simulink model "FullRect_verify"  (R2022b)
settings: Solver=VariableStepAuto  StartTime=0.0  StopTime=0.001  RelTol=1e-3
InitFcn:
  | rng("shuffle");
  | %seed = round(rand(1)*1000);
  | seed = 100;
StopFcn:
  | writematrix(out.input, "C:\Users\dmesenge\Documents\School\PattRecNN\Project\models\FullRect_test_inputs.csv")
  | writematrix(out.actual, "C:\Users\dmesenge\Documents\School\PattRecNN\Project\models\FullRect_test_outputs.csv")
libraries: fl_lib x4, nesl_utility x3, simulink x2, ee_lib x1
settings Model: Creator=dmesenge  LastModifiedBy=dmesenge

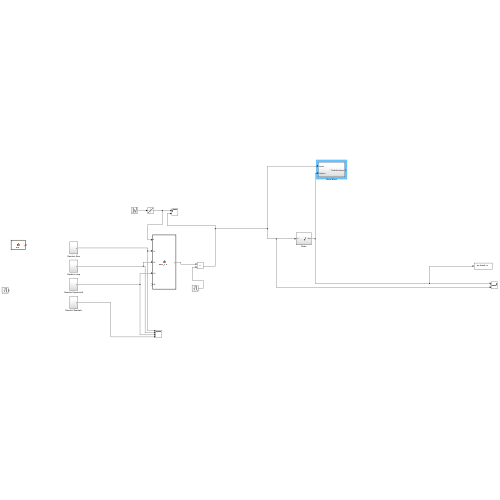
[thumbnail: Simulink's stored preview of the top-level diagram]
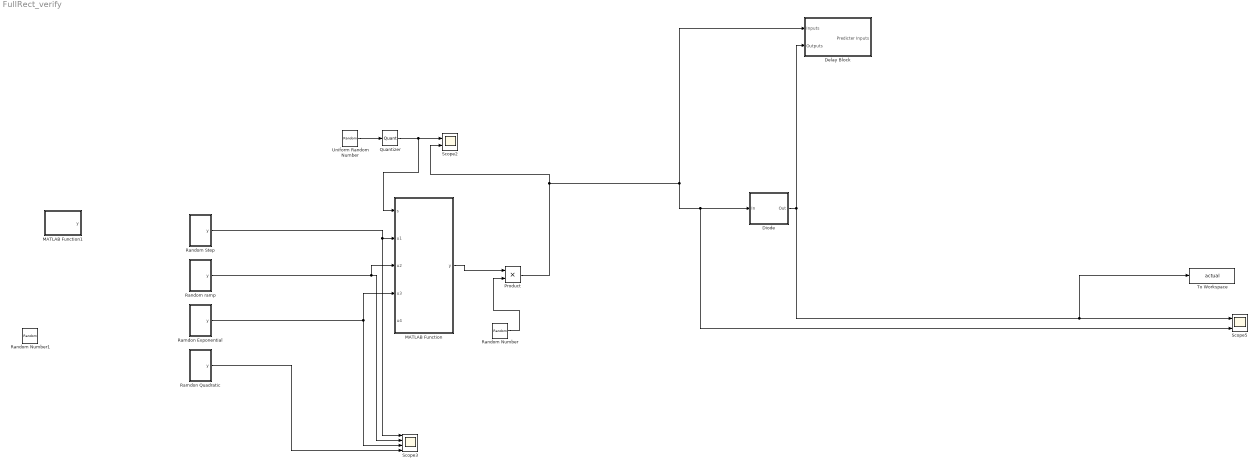
== system FullRect_verify ==
  Delay Block : Subsystem
  Diode : Subsystem
  MATLAB Function : MATLAB Function  TreatAsAtomicUnit=on
  MATLAB Function1 : MATLAB Function  TreatAsAtomicUnit=on
  Product : Product
  Quantizer : Quantizer  QuantizationInterval=1
  Ramdon Exponential : Subsystem
  Ramdon Quadratic : Subsystem
  Random Number : RandomNumber  SampleTime=0.0001
  Random Number1 : RandomNumber  SampleTime=0.00000001
  Random Step : Subsystem
  Random ramp : Subsystem
  Scope2 : Scope  NumInputPorts=2
  Scope3 : Scope  NumInputPorts=4
  Scope5 : Scope  NumInputPorts=3
  To Workspace : ToWorkspace  VariableName=actual  SampleTime=-1
  Uniform Random Number : UniformRandomNumber  Minimum=1  Maximum=4  SampleTime=0.00001
  wires:
  Quantizer/1 -> MATLAB Function/1(s), Scope2/1
  Ramdon Quadratic/1(y) -> Scope3/4
  Random Number/1 -> Product/2
  Random Step/1(y) -> Scope3/1, MATLAB Function/2(u1)
  Ramdon Exponential/1(y) -> Scope3/3, MATLAB Function/4(u3)
  MATLAB Function/1(y) -> Product/1
  Random ramp/1(y) -> MATLAB Function/3(u2), Scope3/2
  Uniform Random Number/1 -> Quantizer/1
  Product/1 -> Delay Block/1(Inputs), Diode/1(In), Scope5/3, Scope2/2
  Diode/1(Out) -> Delay Block/2(Outputs), To Workspace/1, Scope5/1

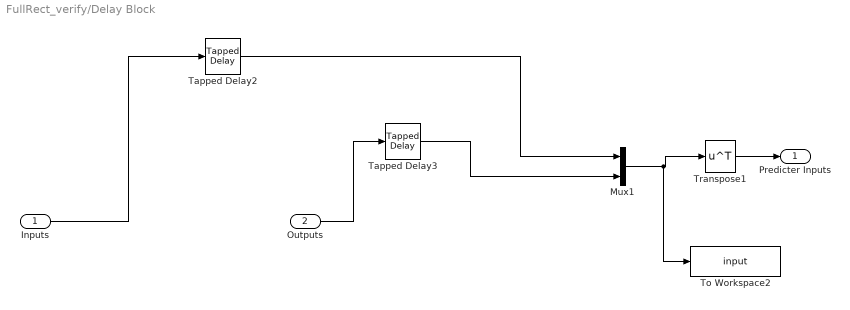
== system FullRect_verify/Delay Block ==
  Inputs : Inport
  Outputs : Inport  Port=2
  Mux1 : Mux  Inputs=2
  Tapped Delay2 : simulink/Discrete/Tapped Delay  vinit=0.0  samptime=-1  NumDelays=9  DelayOrder=Newest  includeCurrent=on
  Tapped Delay3 : simulink/Discrete/Tapped Delay  vinit=0.0  samptime=-1  NumDelays=9  DelayOrder=Newest  includeCurrent=on
  To Workspace2 : ToWorkspace  VariableName=input  SampleTime=-1
  Transpose1 : Math  Operator=transpose
  Predicter Inputs : Outport
  wires:
  Mux1/1 -> To Workspace2/1, Transpose1/1
  Tapped Delay2/1 -> Mux1/1
  Inputs/1 -> Tapped Delay2/1
  Tapped Delay3/1 -> Mux1/2
  Outputs/1 -> Tapped Delay3/1
  Transpose1/1 -> Predicter Inputs/1

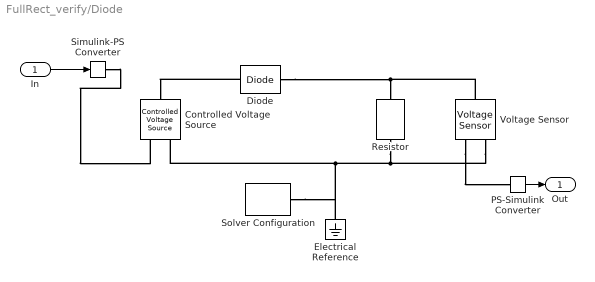
== system FullRect_verify/Diode ==
  In : Inport
  Controlled Voltage Source : fl_lib/Electrical/Electrical Sources/Controlled Voltage Source
  Diode : ee_lib/Semiconductors & Converters/Diode  ModelType=ee.enum.diode.modelType.pwl  TableType=ee.enum.diode.tableType.IfMat  IfMat=[.07, .12, .19, 1.75, 4.24, 7.32, 11.2; .16, .3, .72, 2.14, 5.02, 8.35, 13.12] A  VfMat=[.9, 1.15, 1.25, 1.5, 1.75, 2.17, 2.6, 2.85; .58, .68, .75, 1.1, 1.38, 1.77, 2.27, 2.7] V  TjVec=[25, 125] degC  VfVec=[.5, .7, .9, 1.3, 1.7, 2.1, 2.5] V  IfVec=[.1, .2, .5, 1, 2, 4, 7, 10] A  Vf=0.6 V  Ron=0.3 Ohm  Goff=1e-8 S  prmExp=ee.enum.diode.expParam.useTwo  I12=[.0137, .545] A  V12=[.6, .7] V  RS=0 Ohm  Tmeas=25 degC  IS=1e-12 A  ec=1  I1=0.0137 A  V1=0.6 V  N_series=1  N_parallel=1  Rz=0.3 Ohm  BV=inf V  C_param=ee.enum.diode.capParam.fixed  CJ=0 pF  CJ0=5 pF  Vvec=[.1, 10, 100] V  Cvec=[3.5, 1, .4] pF  VJ=1 V  Mgrad=0.5  FC=0.5  Q_param=ee.enum.diode.recoveryParam.off  iRM=-7.15 A  iF=4 A  didt=-750 A/us  trr_factor=3  trr=115 ns  Qrr=150 nA*s  Vr=-600 V  Ls=150 nH  Erec=0.03 J  TT=50 ns  tau=100 ns  T_param=ee.enum.diode.temperatureParam.off  Tdevice=25 degC  I1_T2=0.245 A  V1_T2=0.5 V  IS_T2=1.25e-7 A  Tmeas2=125 degC  XTI_param=ee.enum.diode.xtiParam.pn  XTI=3  EG_param=ee.enum.diode.egapParam.material_si  EG=1.11 eV  dBVdT=0 V/K  enable_faults=simscape.enum.onoff.off  fault_action=simscape.enum.assert.action.none  fault_types=ee.enum.diode.faults.open  tau_fault=1e-3 s  IfMat_faulted=[.07, .12, .19, 1.75, 4.24, 7.32, 11.2; .16, .3, .72, 2.14, 4.02, 6.35, 9.12] A  VfMat_faulted=[.9, 1.15, 1.25, 1.5, 1.75, 2.17, 2.6, 2.85; .58, .68, .75, 1.1, 1.38, 1.77, 2.27, 2.7] V  VfVec_faulted=[.5, .7, .9, 1.3, 1.7, 2.1, 2.5] V  IfVec_faulted=[.1, .2, .5, 1, 2, 4, 7, 10] A  Ropen_faulted=1000 Ohm  Gshort_faulted=1000 1/Ohm  Vf_faulted=0.6 V  Ron_faulted=0.3 Ohm  Goff_faulted=1e-8 S  I12_faulted=[.0137, .545] A  V12_faulted=[.6, .7] V  IS_faulted=1e-12 A  ec_faulted=1  I1_faulted=0.0137 A  V1_faulted=0.6 V  RS_faulted=0 Ohm  Rz_faulted=0.3 Ohm  BV_faulted=inf V  Cscale_faulted=100  enable_temporal_fault=simscape.enum.onoff.off  t_fault=inf s  enable_behavioral_fault=simscape.enum.onoff.off  max_permissible_voltage=inf V  n_fail_on_voltage=1  max_permissible_current=inf A  t_fail_on_current=1 s  max_permissible_dVdt=inf V/s  enable_fault_input=simscape.enum.onoff.off  i_specify=off  i_priority=None  i=0 A  i_nominal_specify=off  i_nominal_unit=A  i_nominal_value=1  v_specify=off  v_priority=None  v=0 V  v_nominal_specify=off  v_nominal_unit=V  v_nominal_value=1  v_capacitor_specify=off  v_capacitor_priority=None  v_capacitor=0 V  v_capacitor_nominal_specify=off  v_capacitor_nominal_unit=V  v_capacitor_nominal_value=1  i_diode_specify=off  i_diode_priority=None  i_diode=0 A  i_diode_nominal_specify=off  i_diode_nominal_unit=A  i_diode_nominal_value=1  v_diode_specify=off  v_diode_priority=None  v_diode=0 V  v_diode_nominal_specify=off  v_diode_nominal_unit=V  v_diode_nominal_value=1  i_capacitor_specify=off  i_capacitor_priority=None  i_capacitor=0 A  i_capacitor_nominal_specify=off  i_capacitor_nominal_unit=A  i_capacitor_nominal_value=1  power_dissipated_specify=off  power_dissipated_priority=None  power_dissipated=0 W  power_dissipated_nominal_specify=off  power_dissipated_nominal_unit=W  power_dissipated_nominal_value=1  fidelity_level=ee.enum.diode.fidelity.includeChargeDyn  rec_loss_model=ee.enum.diode.reverseRecoveryModel.fixed  ErecVal=0 J  ErecMat=zeros(2, 3) J  TjrecVec=[298.15, 398.15] K  IfrecVec=[.1, 1, 10] A  VrecVal=10 V  tFilter=1 / 1000 / 100 s  max_permissible_temperature=inf K  t_fail_on_temperature=1 s  thermal_network_parameterization=ee.enum.thermalNetworkTopology.junctionCase  Rth=[0, 10] K/W  Rth_Cauer=[1, 3, 10] K/W  Rth_Foster=[4, 6] K/W  thermal_mass_parameterization=ee.enum.thermalNetwork.timeconstant  thermal_mass=[0, 1] J/K  thermal_mass_Cauer=[.1, .3, 1] J/K  thermal_mass_Foster=[1.5, 3] J/K  thermal_time_constant=[0, 10] s  thermal_time_constant_Cauer=[1, 3, 10] s  thermal_time_constant_Foster=[6, 18] s  thermal_mass_initial_temperatures=[25, 25] degC  thermal_mass_initial_temperatures_Cauer=[25, 25, 25] degC  junction_thermal_mass=0.01 J/K  Tvec_initial_Foster=[25, 25, 25, 25] degC  no_thermal_network=0  junction_temperature_specify=off  junction_temperature_priority=None  junction_temperature=25 degC  junction_temperature_nominal_specify=off  junction_temperature_nominal_unit=degC  junction_temperature_nominal_value=1
  Electrical Reference : fl_lib/Electrical/Electrical Elements/Electrical Reference
  PS-Simulink Converter : nesl_utility/PS-Simulink Converter  PhysicalDomain=network_engine_domain  SubClassName=ps_output  LeftPortType=input  RightPortType=output  PseudoPeriodic=off  Frequencies=[]  VectorFormat=inherit  Unit=inherit  AffineConversion=off
  Resistor : fl_lib/Electrical/Electrical Elements/Resistor  R=10000 Ohm  i_specify=off  i_priority=None  i=0 A  i_nominal_specify=off  i_nominal_unit=A  i_nominal_value=1  v_specify=off  v_priority=None  v=0 V  v_nominal_specify=off  v_nominal_unit=V  v_nominal_value=1
  Simulink-PS Converter : nesl_utility/Simulink-PS Converter  PhysicalDomain=network_engine_domain  SubClassName=ps_input  LeftPortType=input  RightPortType=output  PseudoPeriodic=off  Frequencies=[]  NoiseDistribution=none  NoiseParameters=[]  Unit=1  AffineConversion=off  FilteringAndDerivatives=provide  SimscapeFilterOrder=1  InputFilterTimeConstant=0.001  UdotUserProvided=0
  Solver Configuration : nesl_utility/Solver Configuration  PhysicalDomain=network_engine_domain  SubClassName=solver  LeftPortType=input  RightPortType=generic  Tones=[]  Harmonics=[]  SimulateNoise=off  Profile=off  UseLocalSampling=off  EnableSwitchedLinearOptims=on  FrequencyDomain=off  UseCCode=off  RelTol=0.001  AbsTol=0.001  MinStep=1e-09  ToWorkspace=off  RevertToSquareIcSolve=off  NumHomotopyIterations=100  PhasorMode=off  PhasorModeNumHarmonics=1  ConsistencySolver=NEWTON_XTOL_AFTER_FTOL  IndexReductionMethod=DerivativeReplacement  DoDC=off  ResidualTolerance=1e-09  ConsistencyTolSource=GLOBAL  ConsistencyAbsTol=0.001  ConsistencyRelTol=0.001  ConsistencyTolFactor=0.001  UseLocalSolver=off  LocalSolverChoice=NE_BACKWARD_EULER_ADVANCER  ResolveIndetEquations=on  FunctionEvalNumThread=1  LocalSolverSampleTime=0.001  DoFixedCost=off  MaxNonlinIter=3  MaxModeIter=2  ComputeImpulses=off  ImpulseIterations=2  LinearAlgebra=auto  LinearAlgebraNumThread=0  EquationFormulation=NE_TIME_EF  DelaysMemoryBudget=1024  AutomaticFiltering=on  FilteringTimeConstant=0.001  PartitionStorageMethod=AS_NEEDED  PartitionMemoryBudget=1024  PartitionMethod=ROBUST
  Voltage Sensor : fl_lib/Electrical/Electrical Sensors/Voltage Sensor
  Out : Outport
  wires:
  In/1 -> Simulink-PS Converter/1
  PS-Simulink Converter/1 -> Out/1
  connections:
  Voltage Sensor/RConn2 -- Resistor/RConn1 -- Solver Configuration/RConn1 -- Electrical Reference/LConn1 -- Controlled Voltage Source/RConn2
  Diode/LConn1 -- Controlled Voltage Source/LConn1
  Voltage Sensor/RConn1 -- PS-Simulink Converter/LConn1
  Simulink-PS Converter/RConn1 -- Controlled Voltage Source/RConn1
  Diode/RConn1 -- Voltage Sensor/LConn1 -- Resistor/LConn1

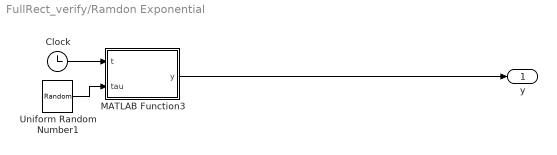
== system FullRect_verify/Ramdon Exponential ==
  Clock : Clock
  MATLAB Function3 : MATLAB Function  TreatAsAtomicUnit=on
  Uniform Random Number1 : UniformRandomNumber  Minimum=-1000  Maximum=1000  Seed=seed  SampleTime=0.00001
  y : Outport
  wires:
  Clock/1 -> MATLAB Function3/1(t)
  Uniform Random Number1/1 -> MATLAB Function3/2(tau)
  MATLAB Function3/1(y) -> y/1

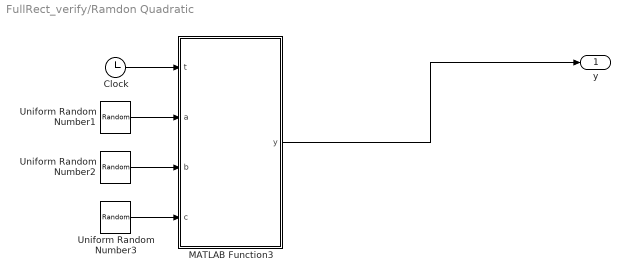
== system FullRect_verify/Ramdon Quadratic ==
  Clock : Clock
  MATLAB Function3 : MATLAB Function  TreatAsAtomicUnit=on
  Uniform Random Number1 : UniformRandomNumber  Minimum=-10  Maximum=10  Seed=seed  SampleTime=0.00001
  Uniform Random Number2 : UniformRandomNumber  Minimum=-100  Maximum=100  Seed=seed  SampleTime=0.00001
  Uniform Random Number3 : UniformRandomNumber  Minimum=-1000  Maximum=1000  Seed=seed  SampleTime=0.00001
  y : Outport
  wires:
  Clock/1 -> MATLAB Function3/1(t)
  Uniform Random Number1/1 -> MATLAB Function3/2(a)
  MATLAB Function3/1(y) -> y/1
  Uniform Random Number3/1 -> MATLAB Function3/4(c)
  Uniform Random Number2/1 -> MATLAB Function3/3(b)

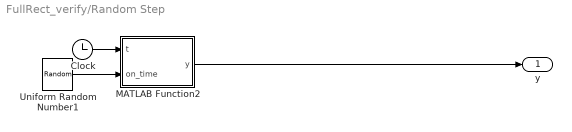
== system FullRect_verify/Random Step ==
  Clock : Clock
  MATLAB Function2 : MATLAB Function  TreatAsAtomicUnit=on
  Uniform Random Number1 : UniformRandomNumber  Minimum=0  Maximum=0.001  Seed=seed  SampleTime=0.00001
  y : Outport
  wires:
  Uniform Random Number1/1 -> MATLAB Function2/2(on_time)
  Clock/1 -> MATLAB Function2/1(t)
  MATLAB Function2/1(y) -> y/1

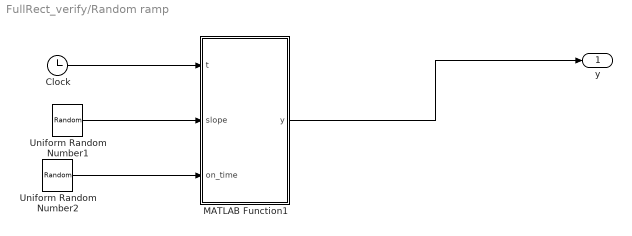
== system FullRect_verify/Random ramp ==
  Clock : Clock
  MATLAB Function1 : MATLAB Function  TreatAsAtomicUnit=on
  Uniform Random Number1 : UniformRandomNumber  Minimum=-10000  Maximum=10000  Seed=seed  SampleTime=0.00001
  Uniform Random Number2 : UniformRandomNumber  Minimum=0  Maximum=0.001  Seed=seed  SampleTime=0.00001
  y : Outport
  wires:
  Uniform Random Number2/1 -> MATLAB Function1/3(on_time)
  Clock/1 -> MATLAB Function1/1(t)
  Uniform Random Number1/1 -> MATLAB Function1/2(slope)
  MATLAB Function1/1(y) -> y/1

== matlab function FullRect_verify/Random ramp/MATLAB Function1 ==
  settings: updateMethod=DISCRETE
  data: t input; y output; slope input; on_time input
function y = rand_ramp(t, slope, on_time)
    %random slope
%     min = -100;
%     max = 100;
%     slope = min+rand()*(max-min);
% 
%     %random on time
%     min = 0;
%     max = 0.001;
%     on_time = min+rand()*(max-min);

    if t < on_time
        r = 0;
    else
        r = slope*t;
    end

y = r;

== matlab function FullRect_verify/MATLAB Function ==
  data: s input; u1 input; y output; u2 input; u3 input; u4 input
function y = mux_4to1(s, u1, u2, u3, u4)
    switch s
       case 1
          r = u1;
       case 2
          r = u2;
       case 3
          r = u3;
       case 4
          r = u4;
       otherwise
          r = u1;
    end

y = r;

== matlab function FullRect_verify/Random Step/MATLAB Function2 ==
  settings: updateMethod=DISCRETE
  data: t input; y output; on_time input
function y = rand_step(t, on_time)

    %random on time
%     min = 0;
%     max = 0.001;
%     on_time = min+rand()*(max-min);

    if t < on_time
        r = 0;
    else
        r = 1;
    end

y = r;

== matlab function FullRect_verify/Ramdon Exponential/MATLAB Function3 ==
  settings: updateMethod=DISCRETE
  data: t input; y output; tau input
function y = rand_exp(t, tau)
    r = exp(t*tau);

y = r;

== matlab function FullRect_verify/Ramdon Quadratic/MATLAB Function3 ==
  settings: updateMethod=DISCRETE
  data: t input; y output; a input; b input; c input
function y = rand_exp(t, a, b, c)
    r = a*t*t + b*t + c;

y = r;

== matlab function FullRect_verify/MATLAB Function1 ==
  data: y output
function y = fcn()
seed = rand(1);
y = rand(1);
